simulink model "AnalyseIMUData"  (R2023a)
settings: Solver=FixedStepAuto  StartTime=0.0  StopTime=inf  RelTol=1e-3  EnableMultiTasking=on
libraries: arduinosensorlib x2
settings Model: ExtModeTrigDuration=2  Creator=The MathWorks, Inc.  LastModifiedBy=Clément
settings SolverCC: MaxZcPerStep=1
settings OptimizationCC: EnhancedBackFolding=on  PassReuseOutputArgsThreshold=0  MaxStackSize=64  OptimizeBlockOrder=speed  DifferentSizesBufferReuse=on  OptimizationCustomize=off
settings DebuggingCC: ParameterPrecisionLossMsg=none  ParameterTunabilityLossMsg=error  UnconnectedInputMsg=warning  UnconnectedOutputMsg=warning  UnconnectedLineMsg=warning
settings HardwareCC: ProdBitPerPointer=32  ProdBitPerSizeT=32  ProdBitPerPtrDiffT=32  ProdLargestAtomicInteger=Long  ProdLargestAtomicFloat=Double  ProdWordSize=32  ProdHWDeviceType=ARM Compatible->ARM Cortex  UseEmbeddedCoderFeatures=off
settings ModelReferenceCC: EnableRefExpFcnMdlSchedulingChecks=on
settings SFSimCC: MATLABDynamicMemAlloc=off
settings RTWCC: Description=Embedded Coder  SystemTargetFile=ert.tlc  HardwareBoard=Arduino MKR1000  TemplateMakefile=ert_default_tmf  Toolchain=Arduino ARM  BuildConfiguration=Faster Runs  DLArmComputeVersion=19.05
settings CodeAppCC: ForceParamTrailComments=on  OperatorAnnotations=on
settings ERTTargetCC: ERTCustomFileBanners=off  SupportContinuousTime=on  SupportNonInlinedSFcns=on  RemoveResetFunc=off  SupportVariableSizeSignals=on  ModelStepFunctionPrototypeControlCompliant=off  ExtModeTransport=3  ExtModeStaticAlloc=on  ExtModeAutomaticAllocSize=off  ExtModeStaticAllocSize=8192  ExtModeMexFile=ext_xcp  ExtModeIntrfLevel=Level2 - Open

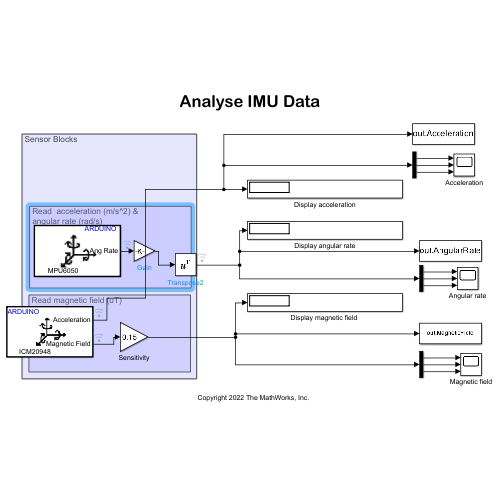
[thumbnail: Simulink's stored preview of the top-level diagram]
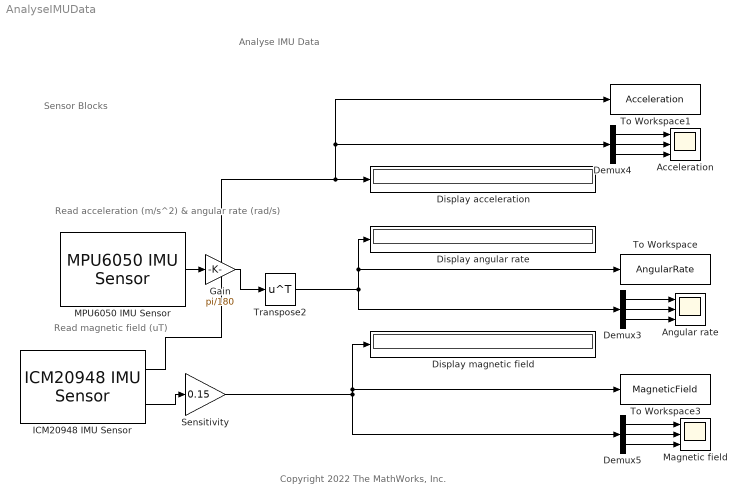
== system AnalyseIMUData ==
  note: Read  acceleration (m/s^2) &
      | angular rate (rad/s)
  note: Read magnetic field (uT)
  note: Sensor Blocks
  note: Copyright 2022 The MathWorks, Inc.
  note: Analyse IMU Data
  Acceleration : Scope  NumInputPorts=3
  Angular rate : Scope  NumInputPorts=3
  Demux3 : Demux  Outputs=3
  Demux4 : Demux  Outputs=3
  Demux5 : Demux  Outputs=3
  Display acceleration : Display
  Display angular rate : Display
  "Display magnetic field " : Display
  Gain : Gain  Gain=pi/180
  ICM20948 IMU Sensor : arduinosensorlib/ICM20948 IMU Sensor  I2CAddress=0x69  BitRate=1000000  EnableDRDY=off  InterruptType=Active high  IsActiveAccel=on  IsActiveGyro=off  IsActiveMag=on  IsActiveTemp=off  IsActiveStatus=off  IsActiveTimeStamp=off  AccelerometerRange=+/-2g  AccelerometerODR=1125  AccelerometerBW=23.9 Hz  GyroscopeRange=+/-250 dps  GyroscopeODR=1125  GyroscopeBW=23.9 Hz  MagnetometerODR=100 Hz  TemperatureBW=34.1 Hz  DataType=double  spf=1  SampleTime=-1  QueueSizeFactor=1
  MPU6050 IMU Sensor : arduinosensorlib/MPU6050 IMU Sensor  SlaveAddress=0x68  Accel=off  AngularRate=on  Temperature=off  Status=off  Timestamp=off  EulerAngles=off  Quat=off  AccelRange=2G  GyroRange=250 dps  DmpOdr=200 Hz  Dlpf=Accelerometer: 184Hz, Gyroscope: 188Hz  spf=1  SampleTime=-1  QueueSizeFactor=1
  Magnetic field : Scope  NumInputPorts=3
  Sensitivity : Gain  Gain=0.15  OutDataTypeStr=double  LockScale=on
  To Workspace : ToWorkspace  VariableName=AngularRate  SampleTime=-1
      settings: Save2DSignal=2-D array (concatenate along first dimension)
  To Workspace1 : ToWorkspace  VariableName=Acceleration  SampleTime=-1
      settings: Save2DSignal=2-D array (concatenate along first dimension)
  To Workspace3 : ToWorkspace  VariableName=MagneticField  SampleTime=-1
      settings: Save2DSignal=2-D array (concatenate along first dimension)
  Transpose2 : Math  Operator=transpose
  wires:
  Demux4/1 -> Acceleration/1
  Demux4/3 -> Acceleration/3
  Demux4/2 -> Acceleration/2
  Demux5/3 -> Magnetic field/3
  Demux5/2 -> Magnetic field/2
  ICM20948 IMU Sensor/1 -> To Workspace1/1, Demux4/1, Display acceleration/1
  Demux5/1 -> Magnetic field/1
  MPU6050 IMU Sensor/1 -> Gain/1
  ICM20948 IMU Sensor/2 -> Sensitivity/1
  Demux3/1 -> Angular rate/1
  Demux3/2 -> Angular rate/2
  Demux3/3 -> Angular rate/3
  Sensitivity/1 -> "Display magnetic field "/1, To Workspace3/1, Demux5/1
  Transpose2/1 -> Display angular rate/1, To Workspace/1, Demux3/1
  Gain/1 -> Transpose2/1
